simulink model "DroneProjectLogicalArchitecture"  (R2023b)
settings: Solver=VariableStepAuto  StartTime=0.0  StopTime=10.0  RelTol=1e-3
settings Model: Creator=lucaerviati  LastModifiedBy=carol
settings OptimizationCC: ReuseModelBlockBuffer=off

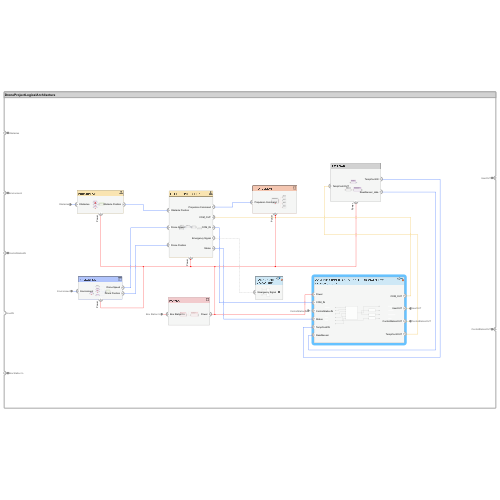
[thumbnail: Simulink's stored preview of the top-level diagram]
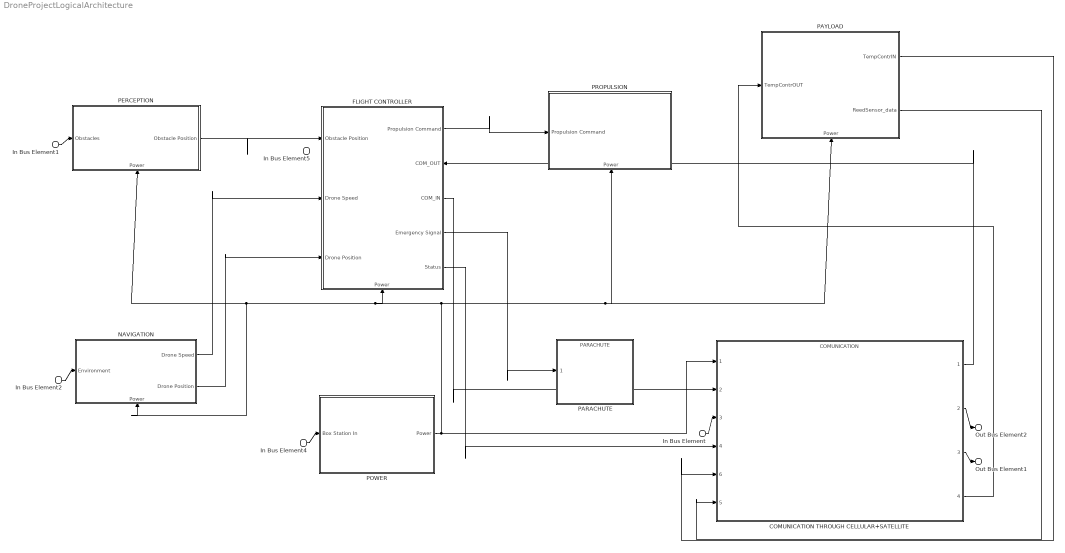
== system DroneProjectLogicalArchitecture ==
  In Bus Element1 : Inport  PortName=Obstacles
  In Bus Element2 : Inport  Port=2  PortName=Environment
  In Bus Element : Inport  Port=3  PortName=ControlStationIN
  In Bus Element5 : Inport  Port=4  PortName=UserIN
  In Bus Element4 : Inport  Port=5  PortName=Box Station In
  COMUNICATION THROUGH CELLULAR+SATELLITE : ModelReference  ModelNameDialog=COMUNICATION  SimulationMode=Normal  ModelReferenceVersion=3.0
      settings: PortSchema="{\"entries\":[{\"content\":{\"headerSize\":38,\"margin\":15,\"minimumSpacing\":25,\"sides\":[{\"content\":{\"connectorIds\":[\"In1\",\"In2\",\"In3\",\"In4\",\"In6\",\"In5\"]},\"type\":\"ConnectorPlacement.EquallySpacedRectSide\",\"uuid\":\"9c17b9ef-2834-4c82-b9e5-e6d3fc257de6\"},{\"content\":{\"connectorIds\":[\"Out1\",\"Out2\",\"Out3\",\"Out4\"],\"side\":\"RIGHT\"},\"type\":\"ConnectorPlacement.EquallySpacedRectSide\",\"uuid\":\"9ecb8183-c057-4821-b5b4-2d9c431b5fb2\"},{\"content\":{\"connectorIds\":[],\"side\":\"TOP\"},\"type\":\"ConnectorPlacement.EquallySpacedRectSide\",\"uuid\":\"bcbced7c-61ac-4e5d-8c11-0c5bb0f95d66\"}]},\"type\":\"ConnectorPlacement.EquallySpacedConnector\",\"uuid\":\"9e4a88fc-7b2c-4c70-8e8f-1bc090782de6\"}],\"packageUris\":[\"http://schema.mathworks.com/mf0/Connector/R2020b\"],\"version\":\"1.0\"}"
  FLIGHT CONTROLLER : Subsystem
      settings: PortSchema="{\"entries\":[{\"content\":{\"headerSize\":26,\"margin\":15,\"minimumSpacing\":25,\"sides\":[{\"content\":{\"connectorIds\":[\"In2\",\"In3\",\"In4\"]},\"type\":\"ConnectorPlacement.EquallySpacedRectSide\",\"uuid\":\"9c17b9ef-2834-4c82-b9e5-e6d3fc257de6\"},{\"content\":{\"connectorIds\":[\"Out1\",\"In1\",\"Out2\",\"Out3\",\"Out4\"],\"side\":\"RIGHT\"},\"type\":\"ConnectorPlacement.EquallySpacedRectSide\",\"uuid\":\"9ecb8183-c057-4821-b5b4-2d9c431b5fb2\"},{\"content\":{\"connectorIds\":[],\"side\":\"TOP\"},\"type\":\"ConnectorPlacement.EquallySpacedRectSide\",\"uuid\":\"bcbced7c-61ac-4e5d-8c11-0c5bb0f95d66\"},{\"content\":{\"connectorIds\":[\"In5\"],\"side\":\"BOTTOM\"},\"type\":\"ConnectorPlacement.EquallySpacedRectSide\",\"uuid\":\"34855c35-e57d-4c91-bde7-679920d0d600\"}]},\"type\":\"ConnectorPlacement.EquallySpacedConnector\",\"uuid\":\"9e4a88fc-7b2c-4c70-8e8f-1bc090782de6\"}],\"packageUris\":[\"http://schema.mathworks.com/mf0/Connector/R2020b\"],\"version\":\"1.0\"}"
  NAVIGATION : Subsystem
      settings: PortSchema="{\"entries\":[{\"content\":{\"headerSize\":26,\"margin\":15,\"minimumSpacing\":25,\"sides\":[{\"content\":{\"connectorIds\":[\"In2\"]},\"type\":\"ConnectorPlacement.EquallySpacedRectSide\",\"uuid\":\"9c17b9ef-2834-4c82-b9e5-e6d3fc257de6\"},{\"content\":{\"connectorIds\":[\"Out1\",\"Out2\"],\"side\":\"RIGHT\"},\"type\":\"ConnectorPlacement.EquallySpacedRectSide\",\"uuid\":\"9ecb8183-c057-4821-b5b4-2d9c431b5fb2\"},{\"content\":{\"side\":\"TOP\"},\"type\":\"ConnectorPlacement.EquallySpacedRectSide\",\"uuid\":\"bcbced7c-61ac-4e5d-8c11-0c5bb0f95d66\"},{\"content\":{\"connectorIds\":[\"In1\"],\"side\":\"BOTTOM\"},\"type\":\"ConnectorPlacement.EquallySpacedRectSide\",\"uuid\":\"d203053f-f656-4182-ab12-058ad919d5d8\"}]},\"type\":\"ConnectorPlacement.EquallySpacedConnector\",\"uuid\":\"9e4a88fc-7b2c-4c70-8e8f-1bc090782de6\"}],\"packageUris\":[\"http://schema.mathworks.com/mf0/Connector/R2020b\"],\"version\":\"1.0\"}"
  PARACHUTE : ModelReference  ModelNameDialog=PARACHUTE  SimulationMode=Normal  ModelReferenceVersion=1.3
      settings: PortSchema="{\"entries\":[{\"content\":{\"headerSize\":38,\"margin\":15,\"minimumSpacing\":25,\"sides\":[{\"content\":{\"connectorIds\":[\"In1\"]},\"type\":\"ConnectorPlacement.EquallySpacedRectSide\",\"uuid\":\"9c17b9ef-2834-4c82-b9e5-e6d3fc257de6\"},{\"content\":{\"connectorIds\":[],\"side\":\"RIGHT\"},\"type\":\"ConnectorPlacement.EquallySpacedRectSide\",\"uuid\":\"9ecb8183-c057-4821-b5b4-2d9c431b5fb2\"},{\"content\":{\"connectorIds\":[],\"side\":\"TOP\"},\"type\":\"ConnectorPlacement.EquallySpacedRectSide\",\"uuid\":\"bcbced7c-61ac-4e5d-8c11-0c5bb0f95d66\"}]},\"type\":\"ConnectorPlacement.EquallySpacedConnector\",\"uuid\":\"9e4a88fc-7b2c-4c70-8e8f-1bc090782de6\"}],\"packageUris\":[\"http://schema.mathworks.com/mf0/Connector/R2020b\"],\"version\":\"1.0\"}"
  PAYLOAD : Subsystem
      settings: PortSchema="{\"entries\":[{\"content\":{\"headerSize\":26,\"margin\":15,\"minimumSpacing\":25,\"sides\":[{\"content\":{\"connectorIds\":[\"In1\"]},\"type\":\"ConnectorPlacement.EquallySpacedRectSide\",\"uuid\":\"9c17b9ef-2834-4c82-b9e5-e6d3fc257de6\"},{\"content\":{\"connectorIds\":[\"Out1\",\"Out2\"],\"side\":\"RIGHT\"},\"type\":\"ConnectorPlacement.EquallySpacedRectSide\",\"uuid\":\"9ecb8183-c057-4821-b5b4-2d9c431b5fb2\"},{\"content\":{\"side\":\"TOP\"},\"type\":\"ConnectorPlacement.EquallySpacedRectSide\",\"uuid\":\"bcbced7c-61ac-4e5d-8c11-0c5bb0f95d66\"},{\"content\":{\"connectorIds\":[\"In2\"],\"side\":\"BOTTOM\"},\"type\":\"ConnectorPlacement.EquallySpacedRectSide\",\"uuid\":\"a0adaaa3-85ad-498a-9bba-69e6a44a934d\"}]},\"type\":\"ConnectorPlacement.EquallySpacedConnector\",\"uuid\":\"9e4a88fc-7b2c-4c70-8e8f-1bc090782de6\"}],\"packageUris\":[\"http://schema.mathworks.com/mf0/Connector/R2020b\"],\"version\":\"1.0\"}"
  PERCEPTION : Subsystem
      settings: PortSchema="{\"entries\":[{\"content\":{\"headerSize\":26,\"margin\":15,\"minimumSpacing\":25,\"sides\":[{\"content\":{\"connectorIds\":[\"In2\"]},\"type\":\"ConnectorPlacement.EquallySpacedRectSide\",\"uuid\":\"9c17b9ef-2834-4c82-b9e5-e6d3fc257de6\"},{\"content\":{\"connectorIds\":[\"Out1\"],\"side\":\"RIGHT\"},\"type\":\"ConnectorPlacement.EquallySpacedRectSide\",\"uuid\":\"9ecb8183-c057-4821-b5b4-2d9c431b5fb2\"},{\"content\":{\"connectorIds\":[],\"side\":\"TOP\"},\"type\":\"ConnectorPlacement.EquallySpacedRectSide\",\"uuid\":\"bcbced7c-61ac-4e5d-8c11-0c5bb0f95d66\"},{\"content\":{\"connectorIds\":[\"In1\"],\"side\":\"BOTTOM\"},\"type\":\"ConnectorPlacement.EquallySpacedRectSide\",\"uuid\":\"015cff9e-64e2-4fe9-90f6-9ce03e119cef\"}]},\"type\":\"ConnectorPlacement.EquallySpacedConnector\",\"uuid\":\"9e4a88fc-7b2c-4c70-8e8f-1bc090782de6\"}],\"packageUris\":[\"http://schema.mathworks.com/mf0/Connector/R2020b\"],\"version\":\"1.0\"}"
  POWER : Subsystem
      settings: PortSchema="{\"entries\":[{\"content\":{\"headerSize\":26,\"margin\":15,\"minimumSpacing\":25,\"sides\":[{\"content\":{\"connectorIds\":[\"In1\"]},\"type\":\"ConnectorPlacement.EquallySpacedRectSide\",\"uuid\":\"9c17b9ef-2834-4c82-b9e5-e6d3fc257de6\"},{\"content\":{\"connectorIds\":[\"Out1\"],\"side\":\"RIGHT\"},\"type\":\"ConnectorPlacement.EquallySpacedRectSide\",\"uuid\":\"9ecb8183-c057-4821-b5b4-2d9c431b5fb2\"},{\"content\":{\"side\":\"TOP\"},\"type\":\"ConnectorPlacement.EquallySpacedRectSide\",\"uuid\":\"bcbced7c-61ac-4e5d-8c11-0c5bb0f95d66\"}]},\"type\":\"ConnectorPlacement.EquallySpacedConnector\",\"uuid\":\"9e4a88fc-7b2c-4c70-8e8f-1bc090782de6\"}],\"packageUris\":[\"http://schema.mathworks.com/mf0/Connector/R2020b\"],\"version\":\"1.0\"}"
  PROPULSION : Subsystem
      settings: PortSchema="{\"entries\":[{\"content\":{\"headerSize\":26,\"margin\":15,\"minimumSpacing\":25,\"sides\":[{\"content\":{\"connectorIds\":[\"In1\"]},\"type\":\"ConnectorPlacement.EquallySpacedRectSide\",\"uuid\":\"9c17b9ef-2834-4c82-b9e5-e6d3fc257de6\"},{\"content\":{\"connectorIds\":[],\"side\":\"RIGHT\"},\"type\":\"ConnectorPlacement.EquallySpacedRectSide\",\"uuid\":\"9ecb8183-c057-4821-b5b4-2d9c431b5fb2\"},{\"content\":{\"connectorIds\":[],\"side\":\"TOP\"},\"type\":\"ConnectorPlacement.EquallySpacedRectSide\",\"uuid\":\"bcbced7c-61ac-4e5d-8c11-0c5bb0f95d66\"},{\"content\":{\"connectorIds\":[\"In2\"],\"side\":\"BOTTOM\"},\"type\":\"ConnectorPlacement.EquallySpacedRectSide\",\"uuid\":\"da01104d-be29-4d48-95e6-05791a72933c\"}]},\"type\":\"ConnectorPlacement.EquallySpacedConnector\",\"uuid\":\"9e4a88fc-7b2c-4c70-8e8f-1bc090782de6\"}],\"packageUris\":[\"http://schema.mathworks.com/mf0/Connector/R2020b\"],\"version\":\"1.0\"}"
  Out Bus Element2 : Outport  PortName=UserOUT
  Out Bus Element1 : Outport  Port=2  PortName=ControlStationOUT
  wires:
  In Bus Element1/1 -> PERCEPTION/2(Obstacles)
  In Bus Element4/1 -> POWER/1(Box Station In)
  POWER/1(Power) -> NAVIGATION/1(Power), PERCEPTION/1(Power), FLIGHT CONTROLLER/5(Power), PROPULSION/2(Power), PAYLOAD/2(Power), COMUNICATION THROUGH CELLULAR+SATELLITE/1
  PERCEPTION/1(Obstacle Position) -> FLIGHT CONTROLLER/2(Obstacle Position)
  In Bus Element2/1 -> NAVIGATION/2(Environment)
  NAVIGATION/1(Drone Speed) -> FLIGHT CONTROLLER/3(Drone Speed)
  NAVIGATION/2(Drone Position) -> FLIGHT CONTROLLER/4(Drone Position)
  FLIGHT CONTROLLER/1(Propulsion Command) -> PROPULSION/1(Propulsion Command)
  FLIGHT CONTROLLER/2(COM_IN) -> COMUNICATION THROUGH CELLULAR+SATELLITE/2
  In Bus Element/1 -> COMUNICATION THROUGH CELLULAR+SATELLITE/3
  PAYLOAD/2(ReedSensor_data) -> COMUNICATION THROUGH CELLULAR+SATELLITE/5
  FLIGHT CONTROLLER/4(Status) -> COMUNICATION THROUGH CELLULAR+SATELLITE/4
  PAYLOAD/1(TempContrIN) -> COMUNICATION THROUGH CELLULAR+SATELLITE/6
  COMUNICATION THROUGH CELLULAR+SATELLITE/1 -> FLIGHT CONTROLLER/1(COM_OUT)
  COMUNICATION THROUGH CELLULAR+SATELLITE/3 -> Out Bus Element1/1
  COMUNICATION THROUGH CELLULAR+SATELLITE/4 -> PAYLOAD/1(TempContrOUT)
  COMUNICATION THROUGH CELLULAR+SATELLITE/2 -> Out Bus Element2/1
  FLIGHT CONTROLLER/3(Emergency Signal) -> PARACHUTE/1

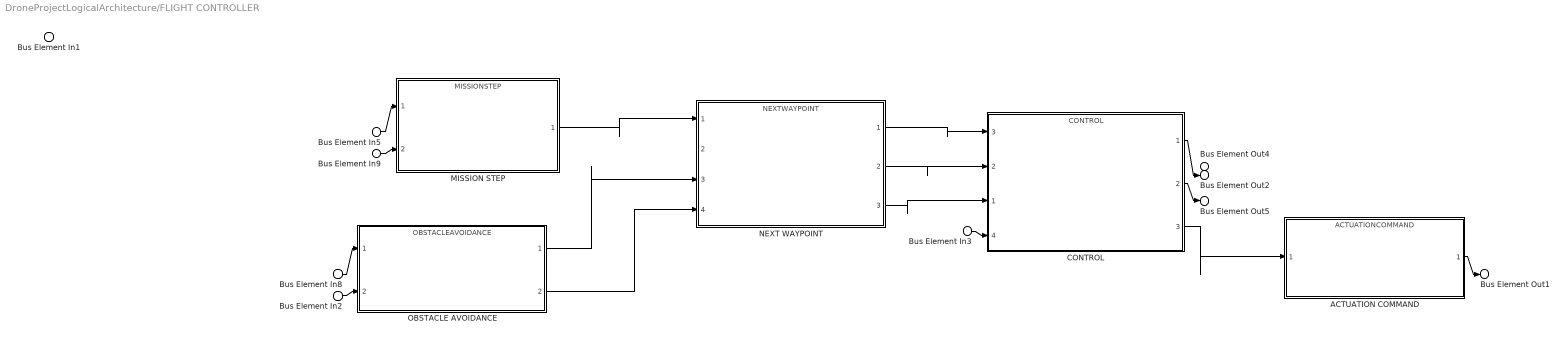
== system DroneProjectLogicalArchitecture/FLIGHT CONTROLLER ==
  Bus Element In5 : Inport  PortName=COM_OUT
  Bus Element In8 : Inport  Port=2  PortName=Obstacle Position
  Bus Element In3 : Inport  Port=3  PortName=Drone Speed
  Bus Element In9 : Inport  Port=4  PortName=Drone Position
  Bus Element In2 : Inport  Port=4  PortName=Drone Position
  Bus Element In1 : Inport  Port=5  PortName=Power
  ACTUATION COMMAND : ModelReference  ModelNameDialog=ACTUATIONCOMMAND  SimulationMode=Normal  ModelReferenceVersion=1.4
      settings: PortSchema="{\"entries\":[{\"content\":{\"headerSize\":38,\"margin\":15,\"minimumSpacing\":25,\"sides\":[{\"content\":{\"connectorIds\":[\"In1\"]},\"type\":\"ConnectorPlacement.EquallySpacedRectSide\",\"uuid\":\"9cca9539-0a36-4124-b22c-ee31f3591a67\"},{\"content\":{\"connectorIds\":[\"Out1\"],\"side\":\"RIGHT\"},\"type\":\"ConnectorPlacement.EquallySpacedRectSide\",\"uuid\":\"eebe1ec1-c849-468b-8863-53f0cc841d23\"},{\"content\":{\"connectorIds\":[],\"side\":\"TOP\"},\"type\":\"ConnectorPlacement.EquallySpacedRectSide\",\"uuid\":\"8f1c4dda-9d7f-4fb5-99d0-4e96ed432329\"}]},\"type\":\"ConnectorPlacement.EquallySpacedConnector\",\"uuid\":\"f7d57f3a-667c-4dfa-8f30-8433699dfbc6\"}],\"packageUris\":[\"http://schema.mathworks.com/mf0/Connector/R2020b\"],\"version\":\"1.0\"}"
  CONTROL : ModelReference  ModelNameDialog=CONTROL  SimulationMode=Normal  ModelReferenceVersion=3.0
      settings: PortSchema="{\"entries\":[{\"content\":{\"headerSize\":38,\"margin\":15,\"minimumSpacing\":25,\"sides\":[{\"content\":{\"connectorIds\":[\"In3\",\"In2\",\"In1\",\"In4\"]},\"type\":\"ConnectorPlacement.EquallySpacedRectSide\",\"uuid\":\"ae43e0f9-cb81-4c7d-a5a1-6ddd261c3f36\"},{\"content\":{\"connectorIds\":[\"Out1\",\"Out2\",\"Out3\"],\"side\":\"RIGHT\"},\"type\":\"ConnectorPlacement.EquallySpacedRectSide\",\"uuid\":\"454013ea-826f-4879-bd33-a0fc10a3e69e\"},{\"content\":{\"side\":\"TOP\"},\"type\":\"ConnectorPlacement.EquallySpacedRectSide\",\"uuid\":\"d045879a-9dfe-4c38-a274-6118b00e003b\"}]},\"type\":\"ConnectorPlacement.EquallySpacedConnector\",\"uuid\":\"e33c714e-0ae2-4a56-8ce0-f9b8de85daa2\"}],\"packageUris\":[\"http://schema.mathworks.com/mf0/Connector/R2020b\"],\"version\":\"1.0\"}"
  MISSION STEP : ModelReference  ModelNameDialog=MISSIONSTEP  SimulationMode=Normal  ModelReferenceVersion=1.5
      settings: PortSchema="{\"entries\":[{\"content\":{\"headerSize\":38,\"margin\":15,\"minimumSpacing\":25,\"sides\":[{\"content\":{\"connectorIds\":[\"In1\",\"In2\"]},\"type\":\"ConnectorPlacement.EquallySpacedRectSide\",\"uuid\":\"ae43e0f9-cb81-4c7d-a5a1-6ddd261c3f36\"},{\"content\":{\"connectorIds\":[\"Out1\"],\"side\":\"RIGHT\"},\"type\":\"ConnectorPlacement.EquallySpacedRectSide\",\"uuid\":\"454013ea-826f-4879-bd33-a0fc10a3e69e\"},{\"content\":{\"connectorIds\":[],\"side\":\"TOP\"},\"type\":\"ConnectorPlacement.EquallySpacedRectSide\",\"uuid\":\"d045879a-9dfe-4c38-a274-6118b00e003b\"}]},\"type\":\"ConnectorPlacement.EquallySpacedConnector\",\"uuid\":\"e33c714e-0ae2-4a56-8ce0-f9b8de85daa2\"}],\"packageUris\":[\"http://schema.mathworks.com/mf0/Connector/R2020b\"],\"version\":\"1.0\"}"
  NEXT WAYPOINT : ModelReference  ModelNameDialog=NEXTWAYPOINT  SimulationMode=Normal  ModelReferenceVersion=1.8
      settings: PortSchema="{\"entries\":[{\"content\":{\"headerSize\":38,\"margin\":15,\"minimumSpacing\":25,\"sides\":[{\"content\":{\"connectorIds\":[\"In1\",\"In2\",\"In3\",\"In4\"]},\"type\":\"ConnectorPlacement.EquallySpacedRectSide\",\"uuid\":\"ae43e0f9-cb81-4c7d-a5a1-6ddd261c3f36\"},{\"content\":{\"connectorIds\":[\"Out1\",\"Out2\",\"Out3\"],\"side\":\"RIGHT\"},\"type\":\"ConnectorPlacement.EquallySpacedRectSide\",\"uuid\":\"454013ea-826f-4879-bd33-a0fc10a3e69e\"},{\"content\":{\"connectorIds\":[],\"side\":\"TOP\"},\"type\":\"ConnectorPlacement.EquallySpacedRectSide\",\"uuid\":\"d045879a-9dfe-4c38-a274-6118b00e003b\"}]},\"type\":\"ConnectorPlacement.EquallySpacedConnector\",\"uuid\":\"e33c714e-0ae2-4a56-8ce0-f9b8de85daa2\"}],\"packageUris\":[\"http://schema.mathworks.com/mf0/Connector/R2020b\"],\"version\":\"1.0\"}"
  OBSTACLE AVOIDANCE : ModelReference  ModelNameDialog=OBSTACLEAVOIDANCE  SimulationMode=Normal  ModelReferenceVersion=3.0
      settings: PortSchema="{\"entries\":[{\"content\":{\"headerSize\":38,\"margin\":15,\"minimumSpacing\":25,\"sides\":[{\"content\":{\"connectorIds\":[\"In1\",\"In2\"]},\"type\":\"ConnectorPlacement.EquallySpacedRectSide\",\"uuid\":\"ae43e0f9-cb81-4c7d-a5a1-6ddd261c3f36\"},{\"content\":{\"connectorIds\":[\"Out1\",\"Out2\"],\"side\":\"RIGHT\"},\"type\":\"ConnectorPlacement.EquallySpacedRectSide\",\"uuid\":\"454013ea-826f-4879-bd33-a0fc10a3e69e\"},{\"content\":{\"connectorIds\":[],\"side\":\"TOP\"},\"type\":\"ConnectorPlacement.EquallySpacedRectSide\",\"uuid\":\"d045879a-9dfe-4c38-a274-6118b00e003b\"}]},\"type\":\"ConnectorPlacement.EquallySpacedConnector\",\"uuid\":\"e33c714e-0ae2-4a56-8ce0-f9b8de85daa2\"}],\"packageUris\":[\"http://schema.mathworks.com/mf0/Connector/R2020b\"],\"version\":\"1.0\"}"
  Bus Element Out1 : Outport  PortName=Propulsion Command
  Bus Element Out4 : Outport  Port=2  PortName=COM_IN
  Bus Element Out2 : Outport  Port=3  PortName=Emergency Signal
  Bus Element Out5 : Outport  Port=4  PortName=Status
  wires:
  Bus Element In2/1 -> OBSTACLE AVOIDANCE/2
  Bus Element In8/1 -> OBSTACLE AVOIDANCE/1
  OBSTACLE AVOIDANCE/1 -> NEXT WAYPOINT/3
  OBSTACLE AVOIDANCE/2 -> NEXT WAYPOINT/4
  Bus Element In9/1 -> MISSION STEP/2
  Bus Element In5/1 -> MISSION STEP/1
  MISSION STEP/1 -> NEXT WAYPOINT/1
  Bus Element In3/1 -> CONTROL/4
  NEXT WAYPOINT/1 -> CONTROL/3
  NEXT WAYPOINT/2 -> CONTROL/2
  NEXT WAYPOINT/3 -> CONTROL/1
  CONTROL/1 -> Bus Element Out2/1
  CONTROL/2 -> Bus Element Out5/1
  CONTROL/3 -> ACTUATION COMMAND/1
  ACTUATION COMMAND/1 -> Bus Element Out1/1

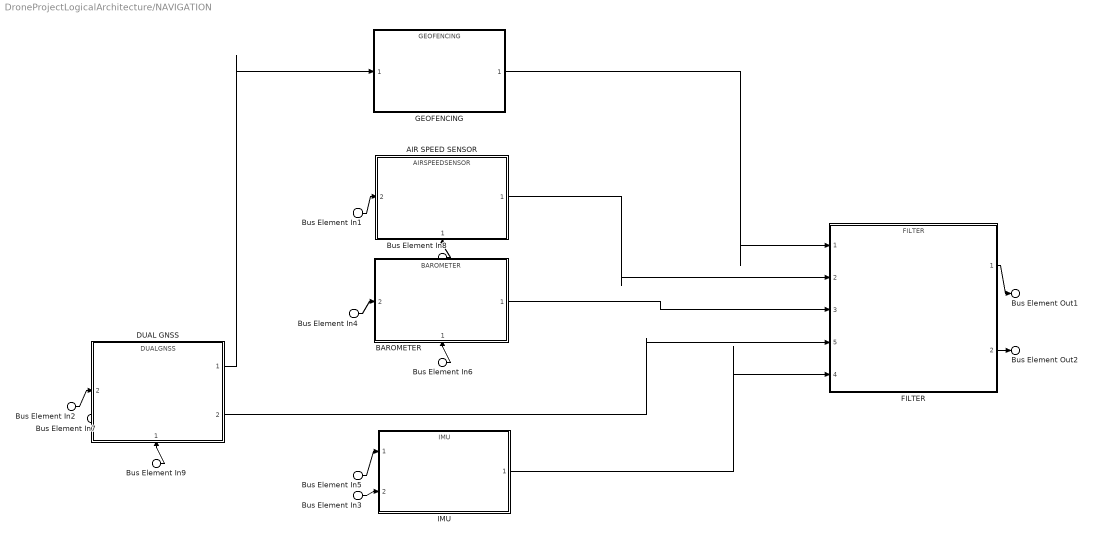
== system DroneProjectLogicalArchitecture/NAVIGATION ==
  Bus Element In{3,6,8..9} (4 alike) : Inport  PortName=Power
  Bus Element In{1..2,4..5,7} (5 alike) : Inport  Port=2  PortName=Environment
  AIR SPEED SENSOR : ModelReference  ModelNameDialog=AIRSPEEDSENSOR  SimulationMode=Normal  ModelReferenceVersion=3.0
      settings: PortSchema="{\"entries\":[{\"content\":{\"headerSize\":38,\"margin\":15,\"minimumSpacing\":25,\"sides\":[{\"content\":{\"connectorIds\":[\"In2\"]},\"type\":\"ConnectorPlacement.EquallySpacedRectSide\",\"uuid\":\"9c17b9ef-2834-4c82-b9e5-e6d3fc257de6\"},{\"content\":{\"connectorIds\":[\"Out1\"],\"side\":\"RIGHT\"},\"type\":\"ConnectorPlacement.EquallySpacedRectSide\",\"uuid\":\"9ecb8183-c057-4821-b5b4-2d9c431b5fb2\"},{\"content\":{\"connectorIds\":[],\"side\":\"TOP\"},\"type\":\"ConnectorPlacement.EquallySpacedRectSide\",\"uuid\":\"bcbced7c-61ac-4e5d-8c11-0c5bb0f95d66\"},{\"content\":{\"connectorIds\":[\"In1\"],\"side\":\"BOTTOM\"},\"type\":\"ConnectorPlacement.EquallySpacedRectSide\",\"uuid\":\"4defc287-ba23-4579-aa3e-e75a55333e42\"}]},\"type\":\"ConnectorPlacement.EquallySpacedConnector\",\"uuid\":\"9e4a88fc-7b2c-4c70-8e8f-1bc090782de6\"}],\"packageUris\":[\"http://schema.mathworks.com/mf0/Connector/R2020b\"],\"version\":\"1.0\"}"
  BAROMETER : ModelReference  ModelNameDialog=BAROMETER  SimulationMode=Normal  ModelReferenceVersion=3.0
      settings: PortSchema="{\"entries\":[{\"content\":{\"headerSize\":38,\"margin\":15,\"minimumSpacing\":25,\"sides\":[{\"content\":{\"connectorIds\":[\"In2\"]},\"type\":\"ConnectorPlacement.EquallySpacedRectSide\",\"uuid\":\"9c17b9ef-2834-4c82-b9e5-e6d3fc257de6\"},{\"content\":{\"connectorIds\":[\"Out1\"],\"side\":\"RIGHT\"},\"type\":\"ConnectorPlacement.EquallySpacedRectSide\",\"uuid\":\"9ecb8183-c057-4821-b5b4-2d9c431b5fb2\"},{\"content\":{\"connectorIds\":[],\"side\":\"TOP\"},\"type\":\"ConnectorPlacement.EquallySpacedRectSide\",\"uuid\":\"bcbced7c-61ac-4e5d-8c11-0c5bb0f95d66\"},{\"content\":{\"connectorIds\":[\"In1\"],\"side\":\"BOTTOM\"},\"type\":\"ConnectorPlacement.EquallySpacedRectSide\",\"uuid\":\"08095248-f23a-4aa7-8f88-7f16feb24103\"}]},\"type\":\"ConnectorPlacement.EquallySpacedConnector\",\"uuid\":\"9e4a88fc-7b2c-4c70-8e8f-1bc090782de6\"}],\"packageUris\":[\"http://schema.mathworks.com/mf0/Connector/R2020b\"],\"version\":\"1.0\"}"
  DUAL GNSS : ModelReference  ModelNameDialog=DUALGNSS  SimulationMode=Normal  ModelReferenceVersion=3.0
      settings: PortSchema="{\"entries\":[{\"content\":{\"headerSize\":38,\"margin\":15,\"minimumSpacing\":25,\"sides\":[{\"content\":{\"connectorIds\":[\"In2\"]},\"type\":\"ConnectorPlacement.EquallySpacedRectSide\",\"uuid\":\"9c17b9ef-2834-4c82-b9e5-e6d3fc257de6\"},{\"content\":{\"connectorIds\":[\"Out1\",\"Out2\"],\"side\":\"RIGHT\"},\"type\":\"ConnectorPlacement.EquallySpacedRectSide\",\"uuid\":\"9ecb8183-c057-4821-b5b4-2d9c431b5fb2\"},{\"content\":{\"connectorIds\":[],\"side\":\"TOP\"},\"type\":\"ConnectorPlacement.EquallySpacedRectSide\",\"uuid\":\"bcbced7c-61ac-4e5d-8c11-0c5bb0f95d66\"},{\"content\":{\"connectorIds\":[\"In1\"],\"side\":\"BOTTOM\"},\"type\":\"ConnectorPlacement.EquallySpacedRectSide\",\"uuid\":\"344d875b-c884-45a5-8f9e-649448aa56aa\"}]},\"type\":\"ConnectorPlacement.EquallySpacedConnector\",\"uuid\":\"9e4a88fc-7b2c-4c70-8e8f-1bc090782de6\"}],\"packageUris\":[\"http://schema.mathworks.com/mf0/Connector/R2020b\"],\"version\":\"1.0\"}"
  FILTER : ModelReference  ModelNameDialog=FILTER  SimulationMode=Normal  ModelReferenceVersion=3.0
      settings: PortSchema="{\"entries\":[{\"content\":{\"headerSize\":38,\"margin\":15,\"minimumSpacing\":25,\"sides\":[{\"content\":{\"connectorIds\":[\"In1\",\"In2\",\"In3\",\"In5\",\"In4\"]},\"type\":\"ConnectorPlacement.EquallySpacedRectSide\",\"uuid\":\"9c17b9ef-2834-4c82-b9e5-e6d3fc257de6\"},{\"content\":{\"connectorIds\":[\"Out1\",\"Out2\"],\"side\":\"RIGHT\"},\"type\":\"ConnectorPlacement.EquallySpacedRectSide\",\"uuid\":\"9ecb8183-c057-4821-b5b4-2d9c431b5fb2\"},{\"content\":{\"connectorIds\":[],\"side\":\"TOP\"},\"type\":\"ConnectorPlacement.EquallySpacedRectSide\",\"uuid\":\"bcbced7c-61ac-4e5d-8c11-0c5bb0f95d66\"}]},\"type\":\"ConnectorPlacement.EquallySpacedConnector\",\"uuid\":\"9e4a88fc-7b2c-4c70-8e8f-1bc090782de6\"}],\"packageUris\":[\"http://schema.mathworks.com/mf0/Connector/R2020b\"],\"version\":\"1.0\"}"
  GEOFENCING : ModelReference  ModelNameDialog=GEOFENCING  SimulationMode=Normal  ModelReferenceVersion=1.3
      settings: PortSchema="{\"entries\":[{\"content\":{\"headerSize\":38,\"margin\":15,\"minimumSpacing\":25,\"sides\":[{\"content\":{\"connectorIds\":[\"In1\"]},\"type\":\"ConnectorPlacement.EquallySpacedRectSide\",\"uuid\":\"9c17b9ef-2834-4c82-b9e5-e6d3fc257de6\"},{\"content\":{\"connectorIds\":[\"Out1\"],\"side\":\"RIGHT\"},\"type\":\"ConnectorPlacement.EquallySpacedRectSide\",\"uuid\":\"9ecb8183-c057-4821-b5b4-2d9c431b5fb2\"},{\"content\":{\"connectorIds\":[],\"side\":\"TOP\"},\"type\":\"ConnectorPlacement.EquallySpacedRectSide\",\"uuid\":\"bcbced7c-61ac-4e5d-8c11-0c5bb0f95d66\"}]},\"type\":\"ConnectorPlacement.EquallySpacedConnector\",\"uuid\":\"9e4a88fc-7b2c-4c70-8e8f-1bc090782de6\"}],\"packageUris\":[\"http://schema.mathworks.com/mf0/Connector/R2020b\"],\"version\":\"1.0\"}"
  IMU : ModelReference  ModelNameDialog=IMU  SimulationMode=Normal  ModelReferenceVersion=3.1
      settings: PortSchema="{\"entries\":[{\"content\":{\"headerSize\":38,\"margin\":15,\"minimumSpacing\":25,\"sides\":[{\"content\":{\"connectorIds\":[\"In1\",\"In2\"]},\"type\":\"ConnectorPlacement.EquallySpacedRectSide\",\"uuid\":\"9c17b9ef-2834-4c82-b9e5-e6d3fc257de6\"},{\"content\":{\"connectorIds\":[\"Out1\"],\"side\":\"RIGHT\"},\"type\":\"ConnectorPlacement.EquallySpacedRectSide\",\"uuid\":\"9ecb8183-c057-4821-b5b4-2d9c431b5fb2\"},{\"content\":{\"connectorIds\":[],\"side\":\"TOP\"},\"type\":\"ConnectorPlacement.EquallySpacedRectSide\",\"uuid\":\"bcbced7c-61ac-4e5d-8c11-0c5bb0f95d66\"}]},\"type\":\"ConnectorPlacement.EquallySpacedConnector\",\"uuid\":\"9e4a88fc-7b2c-4c70-8e8f-1bc090782de6\"}],\"packageUris\":[\"http://schema.mathworks.com/mf0/Connector/R2020b\"],\"version\":\"1.0\"}"
  Bus Element Out1 : Outport  PortName=Drone Speed
  Bus Element Out2 : Outport  Port=2  PortName=Drone Position
  wires:
  DUAL GNSS/2 -> FILTER/5
  FILTER/2 -> Bus Element Out2/1
  FILTER/1 -> Bus Element Out1/1
  DUAL GNSS/1 -> GEOFENCING/1
  GEOFENCING/1 -> FILTER/1
  Bus Element In1/1 -> AIR SPEED SENSOR/2
  Bus Element In8/1 -> AIR SPEED SENSOR/1
  AIR SPEED SENSOR/1 -> FILTER/2
  Bus Element In4/1 -> BAROMETER/2
  Bus Element In6/1 -> BAROMETER/1
  BAROMETER/1 -> FILTER/3
  Bus Element In5/1 -> IMU/1
  Bus Element In3/1 -> IMU/2
  IMU/1 -> FILTER/4
  Bus Element In2/1 -> DUAL GNSS/2
  Bus Element In9/1 -> DUAL GNSS/1

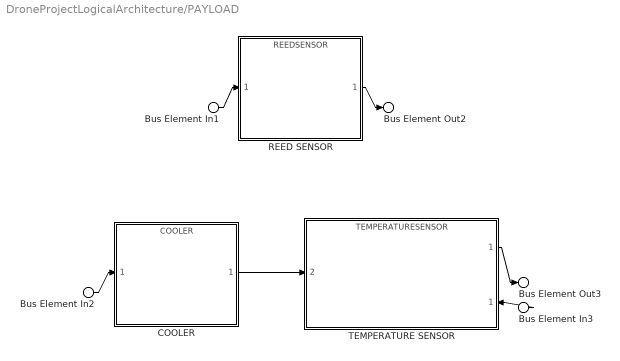
== system DroneProjectLogicalArchitecture/PAYLOAD ==
  Bus Element In3 : Inport  PortName=TempContrOUT
  Bus Element In1 : Inport  Port=2  PortName=Power
  Bus Element In2 : Inport  Port=2  PortName=Power
  COOLER : ModelReference  ModelNameDialog=COOLER  SimulationMode=Normal  ModelReferenceVersion=1.3
      settings: PortSchema="{\"entries\":[{\"content\":{\"headerSize\":38,\"margin\":15,\"minimumSpacing\":25,\"sides\":[{\"content\":{\"connectorIds\":[\"In1\"]},\"type\":\"ConnectorPlacement.EquallySpacedRectSide\",\"uuid\":\"9c17b9ef-2834-4c82-b9e5-e6d3fc257de6\"},{\"content\":{\"connectorIds\":[\"Out1\"],\"side\":\"RIGHT\"},\"type\":\"ConnectorPlacement.EquallySpacedRectSide\",\"uuid\":\"9ecb8183-c057-4821-b5b4-2d9c431b5fb2\"},{\"content\":{\"connectorIds\":[],\"side\":\"TOP\"},\"type\":\"ConnectorPlacement.EquallySpacedRectSide\",\"uuid\":\"bcbced7c-61ac-4e5d-8c11-0c5bb0f95d66\"},{\"content\":{\"connectorIds\":[],\"side\":\"BOTTOM\"},\"type\":\"ConnectorPlacement.EquallySpacedRectSide\",\"uuid\":\"69c8a2c1-8893-417f-9fa0-8793542bfa30\"}]},\"type\":\"ConnectorPlacement.EquallySpacedConnector\",\"uuid\":\"9e4a88fc-7b2c-4c70-8e8f-1bc090782de6\"}],\"packageUris\":[\"http://schema.mathworks.com/mf0/Connector/R2020b\"],\"version\":\"1.0\"}"
  REED SENSOR : ModelReference  ModelNameDialog=REEDSENSOR  SimulationMode=Normal  ModelReferenceVersion=3.0
      settings: PortSchema="{\"entries\":[{\"content\":{\"headerSize\":38,\"margin\":15,\"minimumSpacing\":25,\"sides\":[{\"content\":{\"connectorIds\":[\"In1\"]},\"type\":\"ConnectorPlacement.EquallySpacedRectSide\",\"uuid\":\"9c17b9ef-2834-4c82-b9e5-e6d3fc257de6\"},{\"content\":{\"connectorIds\":[\"Out1\"],\"side\":\"RIGHT\"},\"type\":\"ConnectorPlacement.EquallySpacedRectSide\",\"uuid\":\"9ecb8183-c057-4821-b5b4-2d9c431b5fb2\"},{\"content\":{\"connectorIds\":[],\"side\":\"TOP\"},\"type\":\"ConnectorPlacement.EquallySpacedRectSide\",\"uuid\":\"bcbced7c-61ac-4e5d-8c11-0c5bb0f95d66\"}]},\"type\":\"ConnectorPlacement.EquallySpacedConnector\",\"uuid\":\"9e4a88fc-7b2c-4c70-8e8f-1bc090782de6\"}],\"packageUris\":[\"http://schema.mathworks.com/mf0/Connector/R2020b\"],\"version\":\"1.0\"}"
  "TEMPERATURE SENSOR " : ModelReference  ModelNameDialog=TEMPERATURESENSOR  SimulationMode=Normal  ModelReferenceVersion=3.0
      settings: PortSchema="{\"entries\":[{\"content\":{\"headerSize\":38,\"margin\":15,\"minimumSpacing\":25,\"sides\":[{\"content\":{\"connectorIds\":[\"In2\"]},\"type\":\"ConnectorPlacement.EquallySpacedRectSide\",\"uuid\":\"9c17b9ef-2834-4c82-b9e5-e6d3fc257de6\"},{\"content\":{\"connectorIds\":[\"Out1\",\"In1\"],\"side\":\"RIGHT\"},\"type\":\"ConnectorPlacement.EquallySpacedRectSide\",\"uuid\":\"9ecb8183-c057-4821-b5b4-2d9c431b5fb2\"},{\"content\":{\"connectorIds\":[],\"side\":\"TOP\"},\"type\":\"ConnectorPlacement.EquallySpacedRectSide\",\"uuid\":\"bcbced7c-61ac-4e5d-8c11-0c5bb0f95d66\"}]},\"type\":\"ConnectorPlacement.EquallySpacedConnector\",\"uuid\":\"9e4a88fc-7b2c-4c70-8e8f-1bc090782de6\"}],\"packageUris\":[\"http://schema.mathworks.com/mf0/Connector/R2020b\"],\"version\":\"1.0\"}"
  Bus Element Out3 : Outport  PortName=TempContrIN
  Bus Element Out2 : Outport  Port=2  PortName=ReedSensor_data
  wires:
  Bus Element In1/1 -> REED SENSOR/1
  REED SENSOR/1 -> Bus Element Out2/1
  Bus Element In2/1 -> COOLER/1
  Bus Element In3/1 -> "TEMPERATURE SENSOR "/1
  COOLER/1 -> "TEMPERATURE SENSOR "/2
  "TEMPERATURE SENSOR "/1 -> Bus Element Out3/1

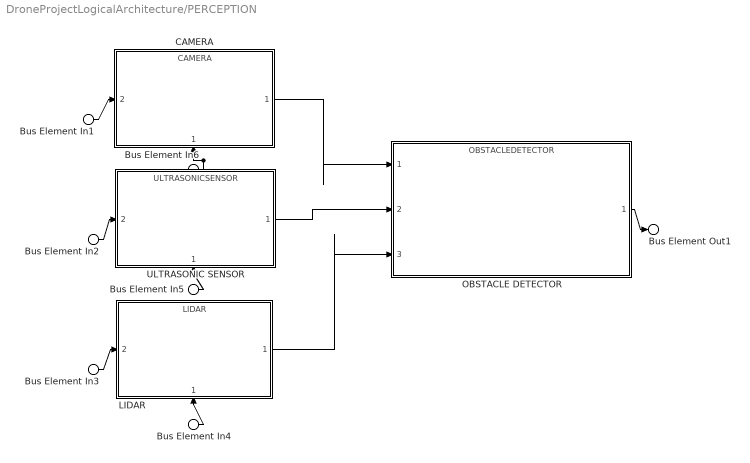
== system DroneProjectLogicalArchitecture/PERCEPTION ==
  Bus Element In4 : Inport  PortName=Power
  Bus Element In5 : Inport  PortName=Power
  Bus Element In6 : Inport  PortName=Power
  Bus Element In2 : Inport  Port=2  PortName=Obstacles
  Bus Element In3 : Inport  Port=2  PortName=Obstacles
  Bus Element In1 : Inport  Port=2  PortName=Obstacles
  CAMERA : ModelReference  ModelNameDialog=CAMERA  SimulationMode=Normal  ModelReferenceVersion=3.0
      settings: PortSchema="{\"entries\":[{\"content\":{\"headerSize\":38,\"margin\":15,\"minimumSpacing\":25,\"sides\":[{\"content\":{\"connectorIds\":[\"In2\"]},\"type\":\"ConnectorPlacement.EquallySpacedRectSide\",\"uuid\":\"9c17b9ef-2834-4c82-b9e5-e6d3fc257de6\"},{\"content\":{\"connectorIds\":[\"Out1\"],\"side\":\"RIGHT\"},\"type\":\"ConnectorPlacement.EquallySpacedRectSide\",\"uuid\":\"9ecb8183-c057-4821-b5b4-2d9c431b5fb2\"},{\"content\":{\"connectorIds\":[],\"side\":\"TOP\"},\"type\":\"ConnectorPlacement.EquallySpacedRectSide\",\"uuid\":\"bcbced7c-61ac-4e5d-8c11-0c5bb0f95d66\"},{\"content\":{\"connectorIds\":[\"In1\"],\"side\":\"BOTTOM\"},\"type\":\"ConnectorPlacement.EquallySpacedRectSide\",\"uuid\":\"6f9eb713-85a4-44f9-8725-fc5d42be12f0\"}]},\"type\":\"ConnectorPlacement.EquallySpacedConnector\",\"uuid\":\"9e4a88fc-7b2c-4c70-8e8f-1bc090782de6\"}],\"packageUris\":[\"http://schema.mathworks.com/mf0/Connector/R2020b\"],\"version\":\"1.0\"}"
  LIDAR : ModelReference  ModelNameDialog=LIDAR  SimulationMode=Normal  ModelReferenceVersion=3.0
      settings: PortSchema="{\"entries\":[{\"content\":{\"headerSize\":38,\"margin\":15,\"minimumSpacing\":25,\"sides\":[{\"content\":{\"connectorIds\":[\"In2\"]},\"type\":\"ConnectorPlacement.EquallySpacedRectSide\",\"uuid\":\"9c17b9ef-2834-4c82-b9e5-e6d3fc257de6\"},{\"content\":{\"connectorIds\":[\"Out1\"],\"side\":\"RIGHT\"},\"type\":\"ConnectorPlacement.EquallySpacedRectSide\",\"uuid\":\"9ecb8183-c057-4821-b5b4-2d9c431b5fb2\"},{\"content\":{\"connectorIds\":[],\"side\":\"TOP\"},\"type\":\"ConnectorPlacement.EquallySpacedRectSide\",\"uuid\":\"bcbced7c-61ac-4e5d-8c11-0c5bb0f95d66\"},{\"content\":{\"connectorIds\":[\"In1\"],\"side\":\"BOTTOM\"},\"type\":\"ConnectorPlacement.EquallySpacedRectSide\",\"uuid\":\"25a9aeed-9787-4c31-8a38-b3b414317afb\"}]},\"type\":\"ConnectorPlacement.EquallySpacedConnector\",\"uuid\":\"9e4a88fc-7b2c-4c70-8e8f-1bc090782de6\"}],\"packageUris\":[\"http://schema.mathworks.com/mf0/Connector/R2020b\"],\"version\":\"1.0\"}"
  OBSTACLE DETECTOR : ModelReference  ModelNameDialog=OBSTACLEDETECTOR  SimulationMode=Normal  ModelReferenceVersion=3.0
      settings: PortSchema="{\"entries\":[{\"content\":{\"headerSize\":38,\"margin\":15,\"minimumSpacing\":25,\"sides\":[{\"content\":{\"connectorIds\":[\"In1\",\"In2\",\"In3\"]},\"type\":\"ConnectorPlacement.EquallySpacedRectSide\",\"uuid\":\"9c17b9ef-2834-4c82-b9e5-e6d3fc257de6\"},{\"content\":{\"connectorIds\":[\"Out1\"],\"side\":\"RIGHT\"},\"type\":\"ConnectorPlacement.EquallySpacedRectSide\",\"uuid\":\"9ecb8183-c057-4821-b5b4-2d9c431b5fb2\"},{\"content\":{\"connectorIds\":[],\"side\":\"TOP\"},\"type\":\"ConnectorPlacement.EquallySpacedRectSide\",\"uuid\":\"bcbced7c-61ac-4e5d-8c11-0c5bb0f95d66\"},{\"content\":{\"connectorIds\":[],\"side\":\"BOTTOM\"},\"type\":\"ConnectorPlacement.EquallySpacedRectSide\",\"uuid\":\"3e107357-9d00-41ed-9250-00f6ff0e10ff\"}]},\"type\":\"ConnectorPlacement.EquallySpacedConnector\",\"uuid\":\"9e4a88fc-7b2c-4c70-8e8f-1bc090782de6\"}],\"packageUris\":[\"http://schema.mathworks.com/mf0/Connector/R2020b\"],\"version\":\"1.0\"}"
  ULTRASONIC SENSOR : ModelReference  ModelNameDialog=ULTRASONICSENSOR  SimulationMode=Normal  ModelReferenceVersion=3.0
      settings: PortSchema="{\"entries\":[{\"content\":{\"headerSize\":38,\"margin\":15,\"minimumSpacing\":25,\"sides\":[{\"content\":{\"connectorIds\":[\"In2\"]},\"type\":\"ConnectorPlacement.EquallySpacedRectSide\",\"uuid\":\"9c17b9ef-2834-4c82-b9e5-e6d3fc257de6\"},{\"content\":{\"connectorIds\":[\"Out1\"],\"side\":\"RIGHT\"},\"type\":\"ConnectorPlacement.EquallySpacedRectSide\",\"uuid\":\"9ecb8183-c057-4821-b5b4-2d9c431b5fb2\"},{\"content\":{\"connectorIds\":[],\"side\":\"TOP\"},\"type\":\"ConnectorPlacement.EquallySpacedRectSide\",\"uuid\":\"bcbced7c-61ac-4e5d-8c11-0c5bb0f95d66\"},{\"content\":{\"connectorIds\":[\"In1\"],\"side\":\"BOTTOM\"},\"type\":\"ConnectorPlacement.EquallySpacedRectSide\",\"uuid\":\"6fa2bf57-cbc6-4fa2-90b4-4f855eb98b37\"}]},\"type\":\"ConnectorPlacement.EquallySpacedConnector\",\"uuid\":\"9e4a88fc-7b2c-4c70-8e8f-1bc090782de6\"}],\"packageUris\":[\"http://schema.mathworks.com/mf0/Connector/R2020b\"],\"version\":\"1.0\"}"
  Bus Element Out1 : Outport  PortName=Obstacle Position
  wires:
  Bus Element In5/1 -> ULTRASONIC SENSOR/1
  Bus Element In2/1 -> ULTRASONIC SENSOR/2
  Bus Element In4/1 -> LIDAR/1
  Bus Element In3/1 -> LIDAR/2
  LIDAR/1 -> OBSTACLE DETECTOR/3
  ULTRASONIC SENSOR/1 -> OBSTACLE DETECTOR/2
  OBSTACLE DETECTOR/1 -> Bus Element Out1/1
  CAMERA/1 -> OBSTACLE DETECTOR/1
  Bus Element In1/1 -> CAMERA/2
  Bus Element In6/1 -> CAMERA/1

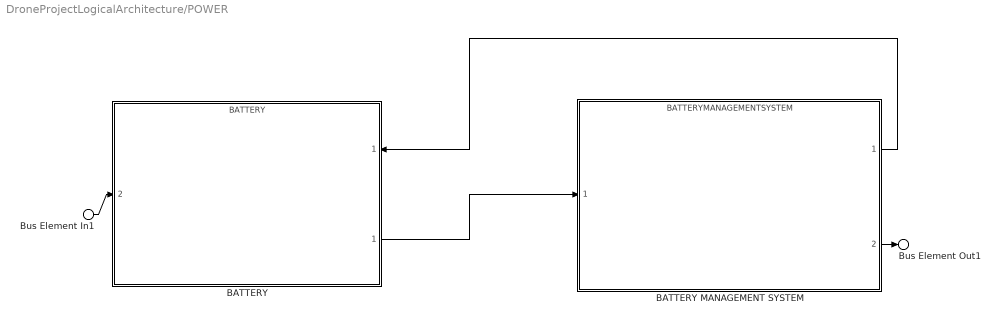
== system DroneProjectLogicalArchitecture/POWER ==
  Bus Element In1 : Inport  PortName=Box Station In
  BATTERY : ModelReference  ModelNameDialog=BATTERY  SimulationMode=Normal  ModelReferenceVersion=3.0
      settings: PortSchema="{\"entries\":[{\"content\":{\"headerSize\":38,\"margin\":15,\"minimumSpacing\":25,\"sides\":[{\"content\":{\"connectorIds\":[\"In2\"]},\"type\":\"ConnectorPlacement.EquallySpacedRectSide\",\"uuid\":\"9c17b9ef-2834-4c82-b9e5-e6d3fc257de6\"},{\"content\":{\"connectorIds\":[\"In1\",\"Out1\"],\"side\":\"RIGHT\"},\"type\":\"ConnectorPlacement.EquallySpacedRectSide\",\"uuid\":\"9ecb8183-c057-4821-b5b4-2d9c431b5fb2\"},{\"content\":{\"connectorIds\":[],\"side\":\"TOP\"},\"type\":\"ConnectorPlacement.EquallySpacedRectSide\",\"uuid\":\"bcbced7c-61ac-4e5d-8c11-0c5bb0f95d66\"}]},\"type\":\"ConnectorPlacement.EquallySpacedConnector\",\"uuid\":\"9e4a88fc-7b2c-4c70-8e8f-1bc090782de6\"}],\"packageUris\":[\"http://schema.mathworks.com/mf0/Connector/R2020b\"],\"version\":\"1.0\"}"
  BATTERY MANAGEMENT SYSTEM : ModelReference  ModelNameDialog=BATTERYMANAGEMENTSYSTEM  SimulationMode=Normal  ModelReferenceVersion=3.1
      settings: PortSchema="{\"entries\":[{\"content\":{\"headerSize\":38,\"margin\":15,\"minimumSpacing\":25,\"sides\":[{\"content\":{\"connectorIds\":[\"In1\"]},\"type\":\"ConnectorPlacement.EquallySpacedRectSide\",\"uuid\":\"9c17b9ef-2834-4c82-b9e5-e6d3fc257de6\"},{\"content\":{\"connectorIds\":[\"Out1\",\"Out2\"],\"side\":\"RIGHT\"},\"type\":\"ConnectorPlacement.EquallySpacedRectSide\",\"uuid\":\"9ecb8183-c057-4821-b5b4-2d9c431b5fb2\"},{\"content\":{\"connectorIds\":[],\"side\":\"TOP\"},\"type\":\"ConnectorPlacement.EquallySpacedRectSide\",\"uuid\":\"bcbced7c-61ac-4e5d-8c11-0c5bb0f95d66\"}]},\"type\":\"ConnectorPlacement.EquallySpacedConnector\",\"uuid\":\"9e4a88fc-7b2c-4c70-8e8f-1bc090782de6\"}],\"packageUris\":[\"http://schema.mathworks.com/mf0/Connector/R2020b\"],\"version\":\"1.0\"}"
  Bus Element Out1 : Outport  PortName=Power
  wires:
  Bus Element In1/1 -> BATTERY/2
  BATTERY/1 -> BATTERY MANAGEMENT SYSTEM/1
  BATTERY MANAGEMENT SYSTEM/2 -> Bus Element Out1/1
  BATTERY MANAGEMENT SYSTEM/1 -> BATTERY/1

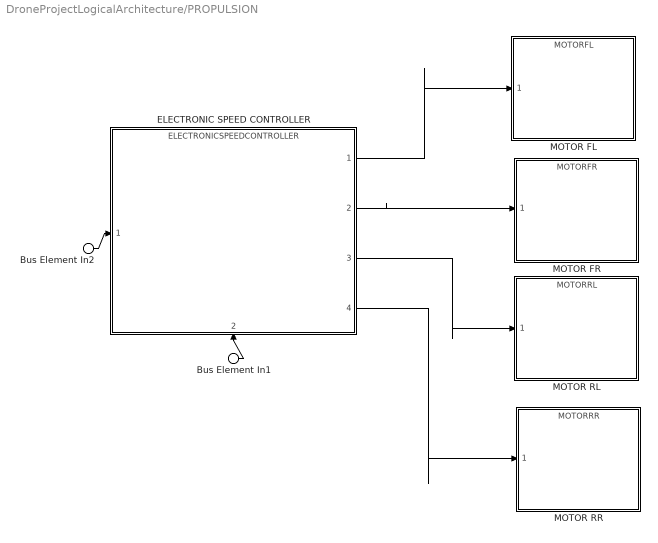
== system DroneProjectLogicalArchitecture/PROPULSION ==
  Bus Element In2 : Inport  PortName=Propulsion Command
  Bus Element In1 : Inport  Port=2  PortName=Power
  ELECTRONIC SPEED CONTROLLER : ModelReference  ModelNameDialog=ELECTRONICSPEEDCONTROLLER  SimulationMode=Normal  ModelReferenceVersion=1.3
      settings: PortSchema="{\"entries\":[{\"content\":{\"headerSize\":38,\"margin\":15,\"minimumSpacing\":25,\"sides\":[{\"content\":{\"connectorIds\":[\"In1\"]},\"type\":\"ConnectorPlacement.EquallySpacedRectSide\",\"uuid\":\"9c17b9ef-2834-4c82-b9e5-e6d3fc257de6\"},{\"content\":{\"connectorIds\":[\"Out1\",\"Out2\",\"Out3\",\"Out4\"],\"side\":\"RIGHT\"},\"type\":\"ConnectorPlacement.EquallySpacedRectSide\",\"uuid\":\"9ecb8183-c057-4821-b5b4-2d9c431b5fb2\"},{\"content\":{\"connectorIds\":[],\"side\":\"TOP\"},\"type\":\"ConnectorPlacement.EquallySpacedRectSide\",\"uuid\":\"bcbced7c-61ac-4e5d-8c11-0c5bb0f95d66\"},{\"content\":{\"connectorIds\":[\"In2\"],\"side\":\"BOTTOM\"},\"type\":\"ConnectorPlacement.EquallySpacedRectSide\",\"uuid\":\"6f56d995-d816-4bf6-84ca-5ab63fa79979\"}]},\"type\":\"ConnectorPlacement.EquallySpacedConnector\",\"uuid\":\"9e4a88fc-7b2c-4c70-8e8f-1bc090782de6\"}],\"packageUris\":[\"http://schema.mathworks.com/mf0/Connector/R2020b\"],\"version\":\"1.0\"}"
  MOTOR FL : ModelReference  ModelNameDialog=MOTORFL  SimulationMode=Normal  ModelReferenceVersion=1.3
      settings: PortSchema="{\"entries\":[{\"content\":{\"headerSize\":38,\"margin\":15,\"minimumSpacing\":25,\"sides\":[{\"content\":{\"connectorIds\":[\"In1\"]},\"type\":\"ConnectorPlacement.EquallySpacedRectSide\",\"uuid\":\"9c17b9ef-2834-4c82-b9e5-e6d3fc257de6\"},{\"content\":{\"connectorIds\":[],\"side\":\"RIGHT\"},\"type\":\"ConnectorPlacement.EquallySpacedRectSide\",\"uuid\":\"9ecb8183-c057-4821-b5b4-2d9c431b5fb2\"},{\"content\":{\"connectorIds\":[],\"side\":\"TOP\"},\"type\":\"ConnectorPlacement.EquallySpacedRectSide\",\"uuid\":\"bcbced7c-61ac-4e5d-8c11-0c5bb0f95d66\"}]},\"type\":\"ConnectorPlacement.EquallySpacedConnector\",\"uuid\":\"9e4a88fc-7b2c-4c70-8e8f-1bc090782de6\"}],\"packageUris\":[\"http://schema.mathworks.com/mf0/Connector/R2020b\"],\"version\":\"1.0\"}"
  MOTOR FR : ModelReference  ModelNameDialog=MOTORFR  SimulationMode=Normal  ModelReferenceVersion=1.3
      settings: PortSchema="{\"entries\":[{\"content\":{\"headerSize\":38,\"margin\":15,\"minimumSpacing\":25,\"sides\":[{\"content\":{\"connectorIds\":[\"In1\"]},\"type\":\"ConnectorPlacement.EquallySpacedRectSide\",\"uuid\":\"9c17b9ef-2834-4c82-b9e5-e6d3fc257de6\"},{\"content\":{\"connectorIds\":[],\"side\":\"RIGHT\"},\"type\":\"ConnectorPlacement.EquallySpacedRectSide\",\"uuid\":\"9ecb8183-c057-4821-b5b4-2d9c431b5fb2\"},{\"content\":{\"connectorIds\":[],\"side\":\"TOP\"},\"type\":\"ConnectorPlacement.EquallySpacedRectSide\",\"uuid\":\"bcbced7c-61ac-4e5d-8c11-0c5bb0f95d66\"}]},\"type\":\"ConnectorPlacement.EquallySpacedConnector\",\"uuid\":\"9e4a88fc-7b2c-4c70-8e8f-1bc090782de6\"}],\"packageUris\":[\"http://schema.mathworks.com/mf0/Connector/R2020b\"],\"version\":\"1.0\"}"
  MOTOR RL : ModelReference  ModelNameDialog=MOTORRL  SimulationMode=Normal  ModelReferenceVersion=1.3
      settings: PortSchema="{\"entries\":[{\"content\":{\"headerSize\":38,\"margin\":15,\"minimumSpacing\":25,\"sides\":[{\"content\":{\"connectorIds\":[\"In1\"]},\"type\":\"ConnectorPlacement.EquallySpacedRectSide\",\"uuid\":\"9c17b9ef-2834-4c82-b9e5-e6d3fc257de6\"},{\"content\":{\"connectorIds\":[],\"side\":\"RIGHT\"},\"type\":\"ConnectorPlacement.EquallySpacedRectSide\",\"uuid\":\"9ecb8183-c057-4821-b5b4-2d9c431b5fb2\"},{\"content\":{\"connectorIds\":[],\"side\":\"TOP\"},\"type\":\"ConnectorPlacement.EquallySpacedRectSide\",\"uuid\":\"bcbced7c-61ac-4e5d-8c11-0c5bb0f95d66\"}]},\"type\":\"ConnectorPlacement.EquallySpacedConnector\",\"uuid\":\"9e4a88fc-7b2c-4c70-8e8f-1bc090782de6\"}],\"packageUris\":[\"http://schema.mathworks.com/mf0/Connector/R2020b\"],\"version\":\"1.0\"}"
  MOTOR RR : ModelReference  ModelNameDialog=MOTORRR  SimulationMode=Normal  ModelReferenceVersion=1.3
      settings: PortSchema="{\"entries\":[{\"content\":{\"headerSize\":38,\"margin\":15,\"minimumSpacing\":25,\"sides\":[{\"content\":{\"connectorIds\":[\"In1\"]},\"type\":\"ConnectorPlacement.EquallySpacedRectSide\",\"uuid\":\"9c17b9ef-2834-4c82-b9e5-e6d3fc257de6\"},{\"content\":{\"connectorIds\":[],\"side\":\"RIGHT\"},\"type\":\"ConnectorPlacement.EquallySpacedRectSide\",\"uuid\":\"9ecb8183-c057-4821-b5b4-2d9c431b5fb2\"},{\"content\":{\"connectorIds\":[],\"side\":\"TOP\"},\"type\":\"ConnectorPlacement.EquallySpacedRectSide\",\"uuid\":\"bcbced7c-61ac-4e5d-8c11-0c5bb0f95d66\"}]},\"type\":\"ConnectorPlacement.EquallySpacedConnector\",\"uuid\":\"9e4a88fc-7b2c-4c70-8e8f-1bc090782de6\"}],\"packageUris\":[\"http://schema.mathworks.com/mf0/Connector/R2020b\"],\"version\":\"1.0\"}"
  wires:
  Bus Element In1/1 -> ELECTRONIC SPEED CONTROLLER/2
  Bus Element In2/1 -> ELECTRONIC SPEED CONTROLLER/1
  ELECTRONIC SPEED CONTROLLER/1 -> MOTOR FL/1
  ELECTRONIC SPEED CONTROLLER/2 -> MOTOR FR/1
  ELECTRONIC SPEED CONTROLLER/3 -> MOTOR RL/1
  ELECTRONIC SPEED CONTROLLER/4 -> MOTOR RR/1
